simulink model "AmbhibiousDroneModel_tilt_mean"  (R2024b)
settings: Solver=FixedStepAuto  StartTime=0.0  StopTime=40  FixedStep=1/3000  RelTol=1e-3
model workspace (MAT data in the model file):
  Cd = 1.63886804e-09
  Ct = 6.43091818e-08
  Ixx = 113600
  Iyy = 113600
  Izz = 22620
  Lx = 0.133
  Ly = 0.1575
  Lz = 0.0132
  h = 0.05
  rho = 1.225
libraries: simulink_extras x10, slpidlib x3, aerolibanimutils x2, shared6dof x1, px4Sensorslib x1
settings Model: Creator=awahm  LastModifiedBy=Micheal Awah
settings RTWCC: GPUComputeCapability=3.5

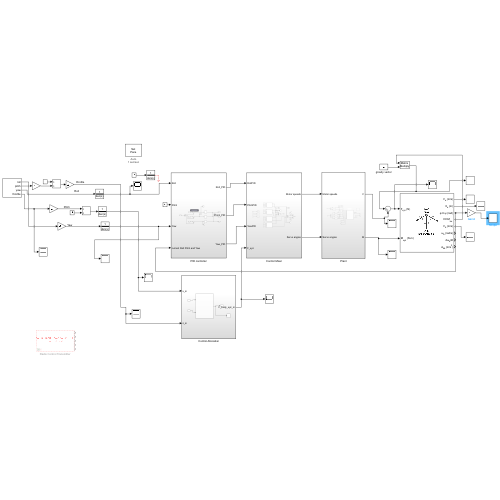
[thumbnail: Simulink's stored preview of the top-level diagram]
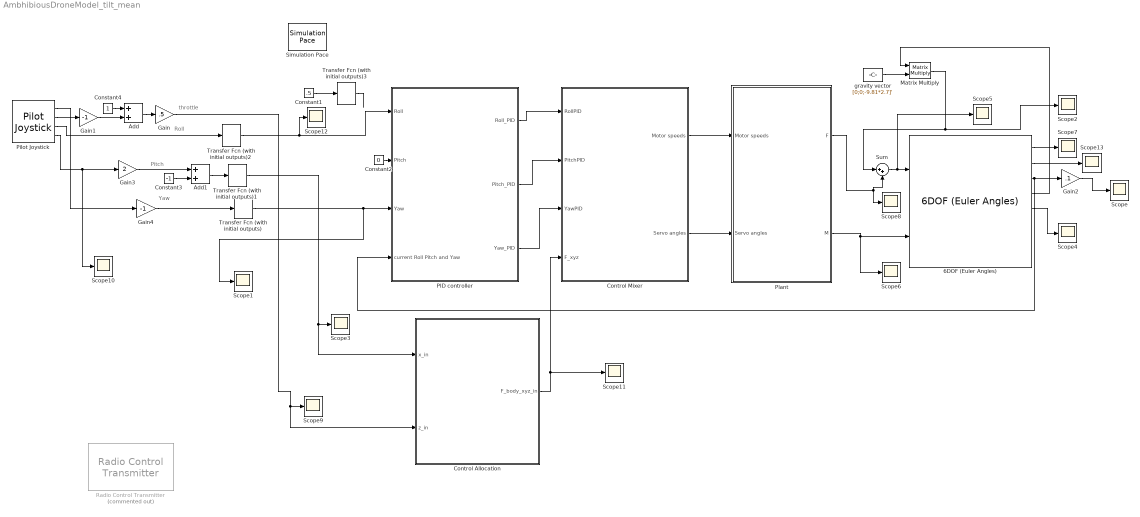
== system AmbhibiousDroneModel_tilt_mean ==
  note: throttle
  note: Roll
  note: Pitch
  note: Yaw
  6DOF (Euler Angles) : shared6dof/6DOF (Euler Angles)  units=Metric (MKS)  mtype=Fixed  rep=Euler Angles  xme_0=[0 0 0]  Vm_0=[0 0 0]  eul_0=[0 0 0]  pm_0=[0 0 0]  mass_0=7.2  mass_e=0.5  mass_f=2.0  inertia=[0.442 0 0;0 0.427 0; 0 0 0.659]  inertia_e=eye(3)  inertia_f=2*eye(3)  k_quat=1.0  vre_flag=on  abi_flag=off  aMode=0  xme_statename=''  Vm_statename=''  eul_statename=''  quat_statename=''  pm_statename=''  mass_statename=''
  Add : Sum
  Add1 : Sum
  Constant1 : Constant  Value=.5
  Constant2 : Constant  Value=0
  Constant3 : Constant  Value=-1
  Constant4 : Constant
  Control Allocation : Subsystem
  Control Mixer : Subsystem
  Gain : Gain  Gain=.5
  Gain1 : Gain  Gain=-1
  Gain2 : Gain  Gain=.1
  Gain3 : Gain  Gain=2
  Gain4 : Gain  Gain=-1
  Matrix Multiply : Product  Multiplication=Matrix(*)
  PID controller : Subsystem
  Pilot Joystick : aerolibanimutils/Pilot Joystick  JoystickID=Joystick1  OutputConfiguration=FourAxis  SampleTime=1/30
  Plant : Subsystem
  Radio Control Transmitter : px4Sensorslib/Radio Control Transmitter  Commented=on  channel1=on  channel2=on  channel3=on  channel4=on  channel5=off  channel6=off  channel7=off  channel8=off  channel_count=off  rssi=off  rc_input_source=off  timestamp_last_signal=off  time_stamp=off  sampleTime=1/250  BlockingMode=off  BlockTimeout=5
  Scope{,1..13} (14 alike) : Scope
  Simulation Pace : aerolibanimutils/Simulation Pace  SimulationPace=1  SleepMode=Auto  OutputPaceError=off  SampleTime=1/300
  Sum : Sum  Inputs=|++
  Transfer Fcn (with initial outputs){,1..3} (4 alike) : simulink_extras/Additional Linear/Transfer Fcn (with initial outputs)  N=[1]  D="[.25  1]"  Y0=0  U0=0
  gravity vector : Constant  Value=[0;0;-9.81*2.7]'
  wires:
  Plant/2(M) -> Scope6/1, 6DOF (Euler Angles)/2
  6DOF (Euler Angles)/4 -> Matrix Multiply/1
  gravity vector/1 -> Matrix Multiply/2
  Sum/1 -> Scope5/1, 6DOF (Euler Angles)/1
  6DOF (Euler Angles)/1 -> Scope7/1
  6DOF (Euler Angles)/5 -> Scope4/1
  Matrix Multiply/1 -> Sum/1, Scope2/1
  Pilot Joystick/1 -> Gain4/1
  PID controller/1(Roll_PID) -> Control Mixer/1(RollPID)
  PID controller/2(Pitch_PID) -> Control Mixer/2(PitchPID)
  PID controller/3(Yaw_PID) -> Control Mixer/3(YawPID)
  Control Mixer/1(Motor speeds) -> Plant/1(Motor speeds)
  Control Mixer/2(Servo angles) -> Plant/2(Servo angles)
  Plant/1(F) -> Sum/2, Scope8/1
  Pilot Joystick/4 -> Gain3/1, Scope10/1
  Pilot Joystick/3 -> Transfer Fcn (with initial outputs)2/1
  Pilot Joystick/2 -> Gain1/1
  Constant4/1 -> Add/1
  Add/1 -> Gain/1
  Gain1/1 -> Add/2
  Constant2/1 -> PID controller/2(Pitch)
  Constant1/1 -> Transfer Fcn (with initial outputs)3/1
  Gain3/1 -> Add1/1
  Constant3/1 -> Add1/2
  Add1/1 -> Transfer Fcn (with initial outputs)1/1
  Gain4/1 -> Transfer Fcn (with initial outputs)/1
  Transfer Fcn (with initial outputs)2/1 -> Scope12/1, PID controller/1(Roll)
  6DOF (Euler Angles)/3 -> Gain2/1, PID controller/4(current Roll Pitch and Yaw)
  Gain/1 -> Scope9/1, Control Allocation/2(z_in)
  Control Allocation/1(F_body_xyz_in) -> Control Mixer/4(F_xyz), Scope11/1
  Transfer Fcn (with initial outputs)/1 -> PID controller/3(Yaw), Scope1/1
  Transfer Fcn (with initial outputs)1/1 -> Control Allocation/1(x_in), Scope3/1
  Transfer Fcn (with initial outputs)3/1 -> ?
  6DOF (Euler Angles)/2 -> Scope13/1
  Gain2/1 -> Scope/1

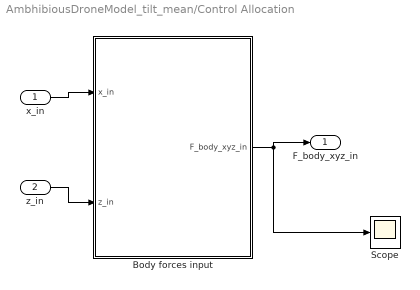
== system AmbhibiousDroneModel_tilt_mean/Control Allocation ==
  x_in : Inport
  z_in : Inport  Port=2
  Body forces input : MATLAB Function  TreatAsAtomicUnit=on
  Scope : Scope
  F_body_xyz_in : Outport
  wires:
  x_in/1 -> Body forces input/1(x_in)
  z_in/1 -> Body forces input/2(z_in)
  Body forces input/1(F_body_xyz_in) -> F_body_xyz_in/1, Scope/1

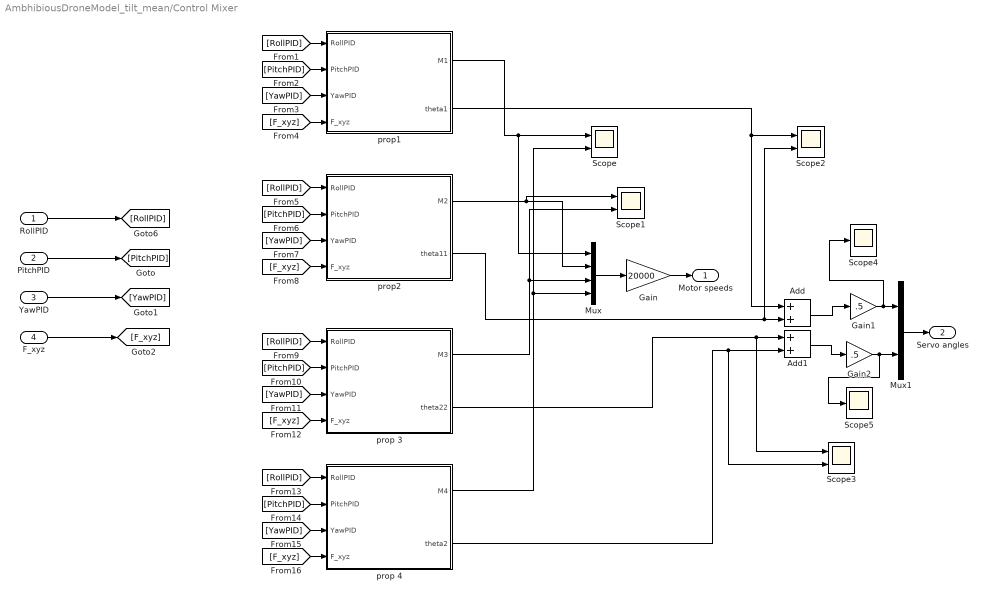
== system AmbhibiousDroneModel_tilt_mean/Control Mixer ==
  RollPID : Inport
  PitchPID : Inport  Port=2
  YawPID : Inport  Port=3
  F_xyz : Inport  Port=4
  Add : Sum
  Add1 : Sum
  Gain : Gain  Gain=20000
  Gain1 : Gain  Gain=.5
  Gain2 : Gain  Gain=.5
  Mux : Mux
  Mux1 : Mux  Inputs=2
  Scope{,1..3} (4 alike) : Scope  NumInputPorts=2
  Scope4 : Scope
  Scope5 : Scope
  prop 3 : Subsystem
  prop 4 : Subsystem
  "prop1 " : Subsystem
  prop2 : Subsystem
  Motor speeds : Outport
  Servo angles : Outport  Port=2
  wires:
  "prop1 "/1(M1) -> Mux/1, Scope/1
  PitchPID/1 -> [PitchPID]
  YawPID/1 -> [YawPID]
  RollPID/1 -> [RollPID]
  [F_xyz] -> "prop1 "/4(F_xyz)
  [YawPID] -> "prop1 "/3(YawPID)
  [PitchPID] -> "prop1 "/2(PitchPID)
  [RollPID] -> "prop1 "/1(RollPID)
  prop2/1(M2) -> Mux/2, Scope1/1
  prop 4/2(theta2) -> Scope3/2, Add1/2
  prop 3/1(M3) -> Scope1/2, Mux/3
  prop 4/1(M4) -> Scope/2, Mux/4
  Mux/1 -> Gain/1
  Mux1/1 -> Servo angles/1
  Gain/1 -> Motor speeds/1
  F_xyz/1 -> [F_xyz]
  [RollPID] -> prop2/1(RollPID)
  [PitchPID] -> prop2/2(PitchPID)
  [YawPID] -> prop2/3(YawPID)
  [F_xyz] -> prop2/4(F_xyz)
  [RollPID] -> prop 3/1(RollPID)
  [PitchPID] -> prop 3/2(PitchPID)
  [YawPID] -> prop 3/3(YawPID)
  [F_xyz] -> prop 3/4(F_xyz)
  [RollPID] -> prop 4/1(RollPID)
  [PitchPID] -> prop 4/2(PitchPID)
  [YawPID] -> prop 4/3(YawPID)
  [F_xyz] -> prop 4/4(F_xyz)
  Gain1/1 -> Scope4/1, Mux1/1
  Gain2/1 -> Scope5/1, Mux1/2
  Add/1 -> Gain1/1
  prop 3/2(theta22) -> Scope3/1, Add1/1
  prop2/2(theta11) -> Scope2/2, Add/2
  "prop1 "/2(theta1) -> Scope2/1, Add/1
  Add1/1 -> Gain2/1

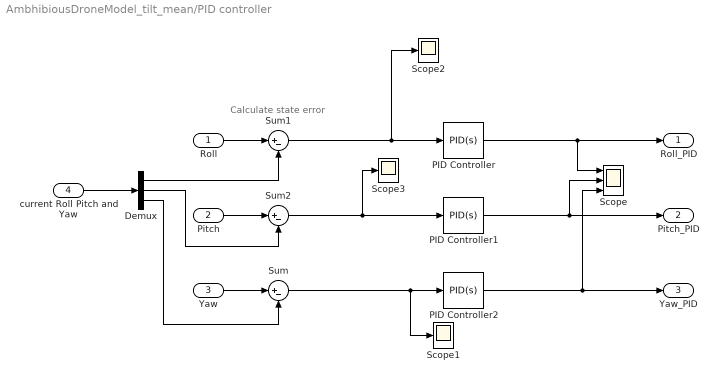
== system AmbhibiousDroneModel_tilt_mean/PID controller ==
  note: Calculate state error
  Roll : Inport
  Pitch : Inport  Port=2
  Yaw : Inport  Port=3
  current Roll Pitch and Yaw : Inport  Port=4
  Demux : Demux  Outputs=3
  PID Controller : slpidlib/PID Controller  Controller=PID  Form=Parallel  TimeDomain=Continuous-time  UseExternalTs=off  SampleTime=-1  IntegratorMethod=Forward Euler  FilterMethod=Forward Euler  ControllerParametersSource=internal  P=.2  I=.3  UseKiTs=off  D=.1  UseExternalDerivativeSource=off  N=100  UseFilter=on  TunerSelectOption=Transfer Function Based (PID Tuner App)  InitialConditionSource=internal  InitialConditionForIntegrator=0  InitialConditionForFilter=0  DifferentiatorICPrevScaledInput=0  ExternalReset=none  TrackingMode=off  Kt=1  LimitOutput=off  SatLimitsSource=internal  UpperSaturationLimit=inf  LowerSaturationLimit=-inf  LinearizeAsGain=on  AntiWindupMode=none  Kb=1  LimitIntegrator=off  UpperIntegratorSaturationLimit=inf  LowerIntegratorSaturationLimit=-inf  POutMin=[]  POutMax=[]  IOutMin=[]  IOutMax=[]  DOutMin=[]  DOutMax=[]  NOutMin=[]  NOutMax=[]  SumOutMin=[]  SumOutMax=[]  SaturationOutMin=[]  SaturationOutMax=[]  PParamMin=[]  PParamMax=[]  IParamMin=[]  IParamMax=[]  DParamMin=[]  DParamMax=[]  NParamMin=[]  NParamMax=[]  KbParamMin=[]  KbParamMax=[]  KtParamMin=[]  KtParamMax=[]  KbOutMin=[]  KbOutMax=[]  KtOutMin=[]  KtOutMax=[]  IntegratorOutMin=[]  IntegratorOutMax=[]  FilterOutMin=[]  FilterOutMax=[]  SumI1OutMin=[]  SumI1OutMax=[]  SumI2OutMin=[]  SumI2OutMax=[]  SumI3OutMin=[]  SumI3OutMax=[]  SumI4OutMin=[]  SumI4OutMax=[]  SumDOutMin=[]  SumDOutMax=[]  DifferentiatorOutMin=[]  DifferentiatorOutMax=[]  FilterDiffOutCoefMin=[]  FilterDiffOutCoefMax=[]  ReciprocalOutMin=[]  ReciprocalOutMax=[]  SumDenOutMin=[]  SumDenOutMax=[]  SumNumOutMin=[]  SumNumOutMax=[]  DivideOutMin=[]  DivideOutMax=[]  UdiffTsProdOutMin=[]  UdiffTsProdOutMax=[]  NTsProdOutMin=[]  NTsProdOutMax=[]  UintegralTsProdOutMin=[]  UintegralTsProdOutMax=[]  UngainTsProdOutMin=[]  UngainTsProdOutMax=[]  ClampingZeroOutDataTypeStr=Inherit: Inherit via back propagation  ClampingZeroOutMin=[]  ClampingZeroOutMax=[]  FilterDenConstantOutDataTypeStr=Inherit: Inherit via back propagation  FilterDenConstantOutMin=[]  FilterDenConstantOutMax=[]  PCopyOutDataTypeStr=Inherit: Inherit via back propagation  PCopyOutMin=[]  PCopyOutMax=[]  NCopyOutDataTypeStr=Inherit: Inherit via back propagation  NCopyOutMin=[]  NCopyOutMax=[]  IntegratorContinuousStateAttributes=''  IntegratorStateMustResolveToSignalObject=off  IntegratorRTWStateStorageClass=Auto  FilterContinuousStateAttributes=''  FilterStateMustResolveToSignalObject=off  FilterRTWStateStorageClass=Auto  ParallelPVariant=InternalParameters  IdealPVariant=Disabled  IVariant=InternalParameters  DVariant=InternalParameters  IntegratorVariant=Continuous  SatVariant=Disabled  AWVariant=Passthrough  PCopyVariant=Disabled  TRVariant=Disabled  FdbkBlocksVariant=Forward  IdealPFdbkVariant=Disabled  SatFdbkVariant=Disabled  DerivativeFilterVariant=ContFilter  NVariant=InternalParameters  NCopyVariant=Disabled  FilterICVariant=InternalICsFilter  IntegratorICVariant=InternalICs  ExternalResetVariant=Disabled  TRSumVariant=Passthrough  SumFdbkVariant=Disabled  SumVariant=Sum_PID  TsampFilterVariant=InternalTs  TsampNgainVariant=Passthrough  TsampIntegralVariant=Disabled_SignalSpec  ExternalSaturationOutDataTypeStr=Inherit: Same as second input  DerivativeSourceVariant=ErrorSignal  PreIntVariant=InternalPreInt
  PID Controller1 : slpidlib/PID Controller  Controller=PID  Form=Parallel  TimeDomain=Continuous-time  UseExternalTs=off  SampleTime=-1  IntegratorMethod=Forward Euler  FilterMethod=Forward Euler  ControllerParametersSource=internal  P=.2  I=.3  UseKiTs=off  D=.1  UseExternalDerivativeSource=off  N=100  UseFilter=on  TunerSelectOption=Transfer Function Based (PID Tuner App)  InitialConditionSource=internal  InitialConditionForIntegrator=0  InitialConditionForFilter=0  DifferentiatorICPrevScaledInput=0  ExternalReset=none  TrackingMode=off  Kt=1  LimitOutput=off  SatLimitsSource=internal  UpperSaturationLimit=inf  LowerSaturationLimit=-inf  LinearizeAsGain=on  AntiWindupMode=none  Kb=1  LimitIntegrator=off  UpperIntegratorSaturationLimit=inf  LowerIntegratorSaturationLimit=-inf  POutMin=[]  POutMax=[]  IOutMin=[]  IOutMax=[]  DOutMin=[]  DOutMax=[]  NOutMin=[]  NOutMax=[]  SumOutMin=[]  SumOutMax=[]  SaturationOutMin=[]  SaturationOutMax=[]  PParamMin=[]  PParamMax=[]  IParamMin=[]  IParamMax=[]  DParamMin=[]  DParamMax=[]  NParamMin=[]  NParamMax=[]  KbParamMin=[]  KbParamMax=[]  KtParamMin=[]  KtParamMax=[]  KbOutMin=[]  KbOutMax=[]  KtOutMin=[]  KtOutMax=[]  IntegratorOutMin=[]  IntegratorOutMax=[]  FilterOutMin=[]  FilterOutMax=[]  SumI1OutMin=[]  SumI1OutMax=[]  SumI2OutMin=[]  SumI2OutMax=[]  SumI3OutMin=[]  SumI3OutMax=[]  SumI4OutMin=[]  SumI4OutMax=[]  SumDOutMin=[]  SumDOutMax=[]  DifferentiatorOutMin=[]  DifferentiatorOutMax=[]  FilterDiffOutCoefMin=[]  FilterDiffOutCoefMax=[]  ReciprocalOutMin=[]  ReciprocalOutMax=[]  SumDenOutMin=[]  SumDenOutMax=[]  SumNumOutMin=[]  SumNumOutMax=[]  DivideOutMin=[]  DivideOutMax=[]  UdiffTsProdOutMin=[]  UdiffTsProdOutMax=[]  NTsProdOutMin=[]  NTsProdOutMax=[]  UintegralTsProdOutMin=[]  UintegralTsProdOutMax=[]  UngainTsProdOutMin=[]  UngainTsProdOutMax=[]  ClampingZeroOutDataTypeStr=Inherit: Inherit via back propagation  ClampingZeroOutMin=[]  ClampingZeroOutMax=[]  FilterDenConstantOutDataTypeStr=Inherit: Inherit via back propagation  FilterDenConstantOutMin=[]  FilterDenConstantOutMax=[]  PCopyOutDataTypeStr=Inherit: Inherit via back propagation  PCopyOutMin=[]  PCopyOutMax=[]  NCopyOutDataTypeStr=Inherit: Inherit via back propagation  NCopyOutMin=[]  NCopyOutMax=[]  IntegratorContinuousStateAttributes=''  IntegratorStateMustResolveToSignalObject=off  IntegratorRTWStateStorageClass=Auto  FilterContinuousStateAttributes=''  FilterStateMustResolveToSignalObject=off  FilterRTWStateStorageClass=Auto  ParallelPVariant=InternalParameters  IdealPVariant=Disabled  IVariant=InternalParameters  DVariant=InternalParameters  IntegratorVariant=Continuous  SatVariant=Disabled  AWVariant=Passthrough  PCopyVariant=Disabled  TRVariant=Disabled  FdbkBlocksVariant=Forward  IdealPFdbkVariant=Disabled  SatFdbkVariant=Disabled  DerivativeFilterVariant=ContFilter  NVariant=InternalParameters  NCopyVariant=Disabled  FilterICVariant=InternalICsFilter  IntegratorICVariant=InternalICs  ExternalResetVariant=Disabled  TRSumVariant=Passthrough  SumFdbkVariant=Disabled  SumVariant=Sum_PID  TsampFilterVariant=InternalTs  TsampNgainVariant=Passthrough  TsampIntegralVariant=Disabled_SignalSpec  ExternalSaturationOutDataTypeStr=Inherit: Same as second input  DerivativeSourceVariant=ErrorSignal  PreIntVariant=InternalPreInt
  PID Controller2 : slpidlib/PID Controller  Controller=PID  Form=Parallel  TimeDomain=Continuous-time  UseExternalTs=off  SampleTime=-1  IntegratorMethod=Forward Euler  FilterMethod=Forward Euler  ControllerParametersSource=internal  P=.2  I=.1  UseKiTs=off  D=.35  UseExternalDerivativeSource=off  N=100  UseFilter=on  TunerSelectOption=Transfer Function Based (PID Tuner App)  InitialConditionSource=internal  InitialConditionForIntegrator=0  InitialConditionForFilter=0  DifferentiatorICPrevScaledInput=0  ExternalReset=none  TrackingMode=off  Kt=1  LimitOutput=off  SatLimitsSource=internal  UpperSaturationLimit=inf  LowerSaturationLimit=-inf  LinearizeAsGain=on  AntiWindupMode=none  Kb=1  LimitIntegrator=off  UpperIntegratorSaturationLimit=inf  LowerIntegratorSaturationLimit=-inf  POutMin=[]  POutMax=[]  IOutMin=[]  IOutMax=[]  DOutMin=[]  DOutMax=[]  NOutMin=[]  NOutMax=[]  SumOutMin=[]  SumOutMax=[]  SaturationOutMin=[]  SaturationOutMax=[]  PParamMin=[]  PParamMax=[]  IParamMin=[]  IParamMax=[]  DParamMin=[]  DParamMax=[]  NParamMin=[]  NParamMax=[]  KbParamMin=[]  KbParamMax=[]  KtParamMin=[]  KtParamMax=[]  KbOutMin=[]  KbOutMax=[]  KtOutMin=[]  KtOutMax=[]  IntegratorOutMin=[]  IntegratorOutMax=[]  FilterOutMin=[]  FilterOutMax=[]  SumI1OutMin=[]  SumI1OutMax=[]  SumI2OutMin=[]  SumI2OutMax=[]  SumI3OutMin=[]  SumI3OutMax=[]  SumI4OutMin=[]  SumI4OutMax=[]  SumDOutMin=[]  SumDOutMax=[]  DifferentiatorOutMin=[]  DifferentiatorOutMax=[]  FilterDiffOutCoefMin=[]  FilterDiffOutCoefMax=[]  ReciprocalOutMin=[]  ReciprocalOutMax=[]  SumDenOutMin=[]  SumDenOutMax=[]  SumNumOutMin=[]  SumNumOutMax=[]  DivideOutMin=[]  DivideOutMax=[]  UdiffTsProdOutMin=[]  UdiffTsProdOutMax=[]  NTsProdOutMin=[]  NTsProdOutMax=[]  UintegralTsProdOutMin=[]  UintegralTsProdOutMax=[]  UngainTsProdOutMin=[]  UngainTsProdOutMax=[]  ClampingZeroOutDataTypeStr=Inherit: Inherit via back propagation  ClampingZeroOutMin=[]  ClampingZeroOutMax=[]  FilterDenConstantOutDataTypeStr=Inherit: Inherit via back propagation  FilterDenConstantOutMin=[]  FilterDenConstantOutMax=[]  PCopyOutDataTypeStr=Inherit: Inherit via back propagation  PCopyOutMin=[]  PCopyOutMax=[]  NCopyOutDataTypeStr=Inherit: Inherit via back propagation  NCopyOutMin=[]  NCopyOutMax=[]  IntegratorContinuousStateAttributes=''  IntegratorStateMustResolveToSignalObject=off  IntegratorRTWStateStorageClass=Auto  FilterContinuousStateAttributes=''  FilterStateMustResolveToSignalObject=off  FilterRTWStateStorageClass=Auto  ParallelPVariant=InternalParameters  IdealPVariant=Disabled  IVariant=InternalParameters  DVariant=InternalParameters  IntegratorVariant=Continuous  SatVariant=Disabled  AWVariant=Passthrough  PCopyVariant=Disabled  TRVariant=Disabled  FdbkBlocksVariant=Forward  IdealPFdbkVariant=Disabled  SatFdbkVariant=Disabled  DerivativeFilterVariant=ContFilter  NVariant=InternalParameters  NCopyVariant=Disabled  FilterICVariant=InternalICsFilter  IntegratorICVariant=InternalICs  ExternalResetVariant=Disabled  TRSumVariant=Passthrough  SumFdbkVariant=Disabled  SumVariant=Sum_PID  TsampFilterVariant=InternalTs  TsampNgainVariant=Passthrough  TsampIntegralVariant=Disabled_SignalSpec  ExternalSaturationOutDataTypeStr=Inherit: Same as second input  DerivativeSourceVariant=ErrorSignal  PreIntVariant=InternalPreInt
  Scope : Scope  NumInputPorts=3
  Scope1 : Scope
  Scope2 : Scope
  Scope3 : Scope
  Sum : Sum  Inputs=|+-
  Sum1 : Sum  Inputs=|+-
  Sum2 : Sum  Inputs=|+-
  Roll_PID : Outport
  Pitch_PID : Outport  Port=2
  Yaw_PID : Outport  Port=3
  wires:
  Demux/3 -> Sum/2
  Demux/2 -> Sum2/2
  Demux/1 -> Sum1/2
  current Roll Pitch and Yaw/1 -> Demux/1
  Sum/1 -> Scope1/1, PID Controller2/1
  Roll/1 -> Sum1/1
  Pitch/1 -> Sum2/1
  Yaw/1 -> Sum/1
  Sum1/1 -> Scope2/1, PID Controller/1
  Sum2/1 -> Scope3/1, PID Controller1/1
  PID Controller/1 -> Roll_PID/1, Scope/1
  PID Controller2/1 -> Yaw_PID/1, Scope/3
  PID Controller1/1 -> Pitch_PID/1, Scope/2

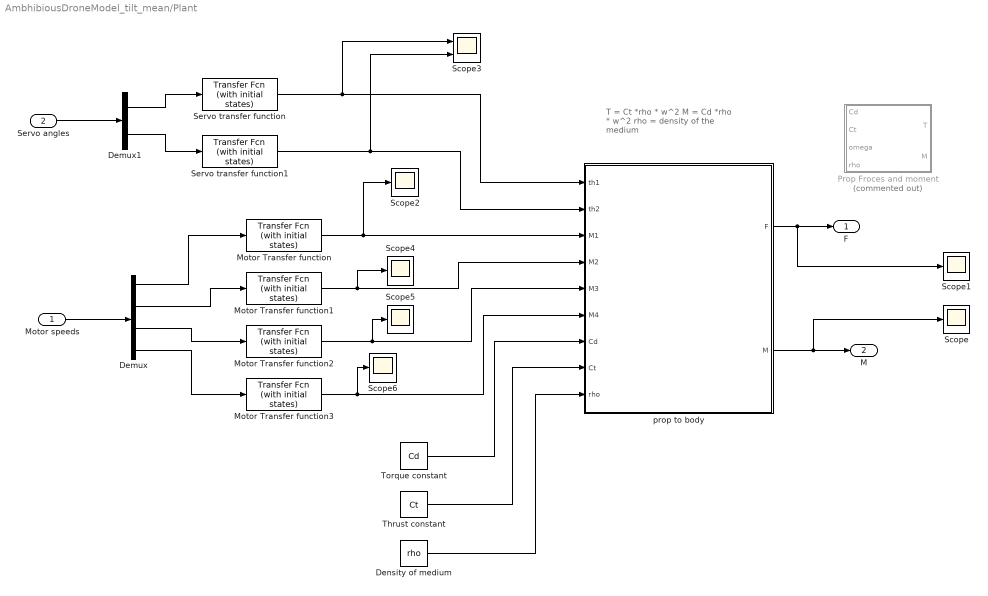
== system AmbhibiousDroneModel_tilt_mean/Plant ==
  note: T = Ct *rho * w^2
      | M = Cd *rho * w^2
      | rho = density of the medium
  Motor speeds : Inport
  Servo angles : Inport  Port=2
  Demux : Demux
  Demux1 : Demux  Outputs=2
  Density of medium : Constant  Value=rho
  Motor Transfer function{,1..3} (4 alike) : simulink_extras/Additional Linear/Transfer Fcn (with initial states)  N=[153.35]  D=[1 20.06 153.35]  X0=0
  Prop Froces and moment : Subsystem  Commented=on
  Scope{,1..2,4..6} (6 alike) : Scope
  Scope3 : Scope  NumInputPorts=2
  Servo transfer function : simulink_extras/Additional Linear/Transfer Fcn (with initial states)  N=[153.35]  D=[1 20.06 153.35]  X0=0
  Servo transfer function1 : simulink_extras/Additional Linear/Transfer Fcn (with initial states)  N=[153.35]  D=[1 20.06 153.35]  X0=0
  Thrust constant : Constant  Value=Ct
  Torque constant : Constant  Value=Cd
  prop to body : MATLAB Function  TreatAsAtomicUnit=on
  F : Outport
  M : Outport  Port=2
  wires:
  Motor speeds/1 -> Demux/1
  Servo angles/1 -> Demux1/1
  Demux/3 -> Motor Transfer function2/1
  Demux/4 -> Motor Transfer function3/1
  Demux1/1 -> Servo transfer function/1
  Demux1/2 -> Servo transfer function1/1
  Demux/1 -> Motor Transfer function/1
  Demux/2 -> Motor Transfer function1/1
  Thrust constant/1 -> prop to body/8(Ct)
  prop to body/1(F) -> Scope1/1, F/1
  Torque constant/1 -> prop to body/7(Cd)
  Motor Transfer function/1 -> Scope2/1, prop to body/3(M1)
  Density of medium/1 -> prop to body/9(rho)
  Motor Transfer function1/1 -> Scope4/1, prop to body/4(M2)
  Motor Transfer function2/1 -> Scope5/1, prop to body/5(M3)
  Motor Transfer function3/1 -> Scope6/1, prop to body/6(M4)
  Servo transfer function1/1 -> Scope3/2, prop to body/2(th2)
  prop to body/2(M) -> Scope/1, M/1
  Servo transfer function/1 -> Scope3/1, prop to body/1(th1)

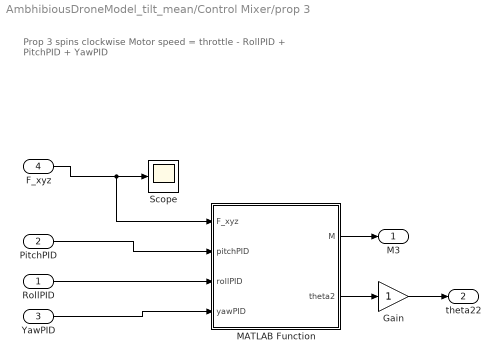
== system AmbhibiousDroneModel_tilt_mean/Control Mixer/prop 3 ==
  note: Prop 3 spins clockwise
      | Motor speed = throttle - RollPID + PitchPID + YawPID
  RollPID : Inport
  PitchPID : Inport  Port=2
  YawPID : Inport  Port=3
  F_xyz : Inport  Port=4
  Gain : Gain
  MATLAB Function : MATLAB Function  TreatAsAtomicUnit=on
  Scope : Scope
  M3 : Outport
  theta22 : Outport  Port=2
  wires:
  YawPID/1 -> MATLAB Function/4(yawPID)
  F_xyz/1 -> MATLAB Function/1(F_xyz), Scope/1
  RollPID/1 -> MATLAB Function/3(rollPID)
  MATLAB Function/1(M) -> M3/1
  MATLAB Function/2(theta2) -> Gain/1
  PitchPID/1 -> MATLAB Function/2(pitchPID)
  Gain/1 -> theta22/1

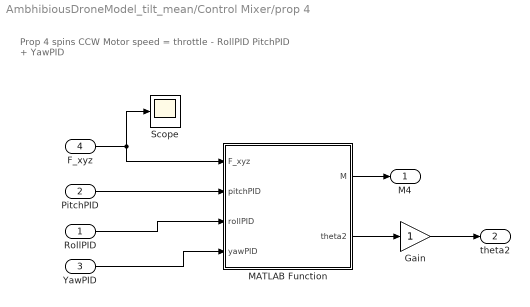
== system AmbhibiousDroneModel_tilt_mean/Control Mixer/prop 4 ==
  note: Prop 4 spins CCW
      | Motor speed = throttle - RollPID   PitchPID + YawPID
  RollPID : Inport
  PitchPID : Inport  Port=2
  YawPID : Inport  Port=3
  F_xyz : Inport  Port=4
  Gain : Gain
  MATLAB Function : MATLAB Function  TreatAsAtomicUnit=on
  Scope : Scope
  M4 : Outport
  theta2 : Outport  Port=2
  wires:
  YawPID/1 -> MATLAB Function/4(yawPID)
  F_xyz/1 -> Scope/1, MATLAB Function/1(F_xyz)
  RollPID/1 -> MATLAB Function/3(rollPID)
  PitchPID/1 -> MATLAB Function/2(pitchPID)
  MATLAB Function/1(M) -> M4/1
  MATLAB Function/2(theta2) -> Gain/1
  Gain/1 -> theta2/1

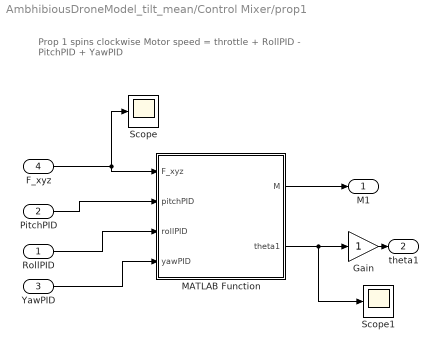
== system AmbhibiousDroneModel_tilt_mean/Control Mixer/prop1  ==
  note: Prop 1 spins clockwise
      | Motor speed = throttle + RollPID - PitchPID + YawPID
  RollPID : Inport
  PitchPID : Inport  Port=2
  YawPID : Inport  Port=3
  F_xyz : Inport  Port=4
  Gain : Gain
  MATLAB Function : MATLAB Function  TreatAsAtomicUnit=on
  Scope : Scope
  Scope1 : Scope
  M1 : Outport
  theta1 : Outport  Port=2
  wires:
  MATLAB Function/2(theta1) -> Scope1/1, Gain/1
  F_xyz/1 -> Scope/1, MATLAB Function/1(F_xyz)
  RollPID/1 -> MATLAB Function/3(rollPID)
  PitchPID/1 -> MATLAB Function/2(pitchPID)
  YawPID/1 -> MATLAB Function/4(yawPID)
  MATLAB Function/1(M) -> M1/1
  Gain/1 -> theta1/1

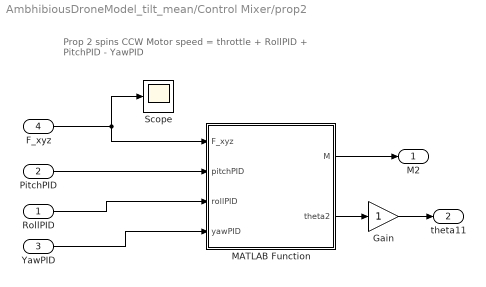
== system AmbhibiousDroneModel_tilt_mean/Control Mixer/prop2 ==
  note: Prop 2 spins CCW
      | Motor speed = throttle + RollPID + PitchPID - YawPID
  RollPID : Inport
  PitchPID : Inport  Port=2
  YawPID : Inport  Port=3
  F_xyz : Inport  Port=4
  Gain : Gain
  MATLAB Function : MATLAB Function  TreatAsAtomicUnit=on
  Scope : Scope
  M2 : Outport
  theta11 : Outport  Port=2
  wires:
  YawPID/1 -> MATLAB Function/4(yawPID)
  F_xyz/1 -> Scope/1, MATLAB Function/1(F_xyz)
  RollPID/1 -> MATLAB Function/3(rollPID)
  PitchPID/1 -> MATLAB Function/2(pitchPID)
  MATLAB Function/1(M) -> M2/1
  MATLAB Function/2(theta2) -> Gain/1
  Gain/1 -> theta11/1

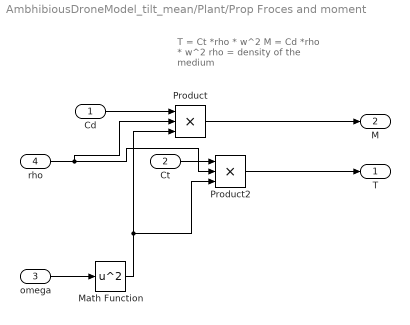
== system AmbhibiousDroneModel_tilt_mean/Plant/Prop Froces and moment ==
  note: T = Ct *rho * w^2
      | M = Cd *rho * w^2
      | rho = density of the medium
  Cd : Inport
  Ct : Inport  Port=2
  omega : Inport  Port=3
  rho : Inport  Port=4
  Math Function : Math  Operator=square
  Product : Product  Inputs=3
  Product2 : Product  Inputs=3
  T : Outport
  M : Outport  Port=2
  wires:
  omega/1 -> Math Function/1
  Ct/1 -> Product2/1
  Product2/1 -> T/1
  Product/1 -> M/1
  Cd/1 -> Product/1
  Math Function/1 -> Product2/3, Product/3
  rho/1 -> Product/2, Product2/2

== matlab function AmbhibiousDroneModel_tilt_mean/Plant/prop to body ==
  data: th1 input; F output; th2 input; M1 input; M2 input; M3 input; M4 input; Cd input; Ct input; rho input; M output
function [F,M] = fcn(th1,th2,M1,M2,M3,M4,Cd,Ct,rho)

T1 = Ct*rho*M1^2;
T2 = Ct*rho*M2^2;
T3 = Ct*rho*M3^2;
T4 = Ct*rho*M4^2;

C = Cd/Ct;

Ly = 0.133;
Lx = 0.1575;
d = -0.0132;

y = [Ly*T1*cos(th1) - Ly*T2*cos(th1) - Ly*T3*cos(th2) + Ly*T4*cos(th2) - C*T1*sin(th1) + C*T2*sin(th1) - C*T3*sin(th2) + C*T4*sin(th2);
     T3*(Lx*cos(th2) + d*sin(th2)) - T2*(Lx*cos(th1) - d*sin(th1)) - T1*(Lx*cos(th1) - d*sin(th1)) + T4*(Lx*cos(th2) + d*sin(th2));
     C*T2*cos(th1) - C*T1*cos(th1) - C*T3*cos(th2) + C*T4*cos(th2) - Ly*T1*sin(th1) + Ly*T2*sin(th1) + Ly*T3*sin(th2) - Ly*T4*sin(th2);
                                                                            T1*sin(th1) + T2*sin(th1) + T3*sin(th2) + T4*sin(th2);
                                                                                                                                0;
                                                                            T1*cos(th1) + T2*cos(th1) + T3*cos(th2) + T4*cos(th2)];
M = y(1:3);
F = y(4:6);

== matlab function AmbhibiousDroneModel_tilt_mean/Control Allocation/Body forces input ==
  data: x_in input; F_body_xyz_in output; z_in input
function F_body_xyz_in = fcn(x_in, z_in)
g = 9.81;
mass = 2.7;
V_cap = [x_in;0;z_in];  
F_body_xyz_in = V_cap;

% if z_in >= 0.5
%     % Define the input range
%     input_min = 0.5;
%     input_max = 1;
% 
%     % Define the output range
%     % output_min = 0;
%     output_max = 20; %making upward vertical acceleration
% 
%     % Map the input value to the output range
%     output_value = ((z_in - input_min) / (input_max - input_min)) * (output_max - output_min) + output_min;
% else
%     % Define the input range
%     input_min = 0;
%     input_max = 0.5;
% 
%     % Define the output range
%     output_min = -5; %max possible downward acceleration
%     output_max = 0;
% 
%     % Map the input value to the output range
%     output_value = ((z_in - input_min) / (input_max - input_min)) * (output_max - output_min) + output_min;
% end
% 
% F_body_xyz_in(3) = F_body_xyz_in(3) + output_value*mass; %adding acceleration due to throttle
% 
% deno = sqrt(F_body_xyz_in(3)^2 + F_body_xyz_in(1)^2);  %to use for norm, not that y-comp is not effective
% F_body_xyz_in = F_body_xyz_in/deno;  %normalizing

== matlab function AmbhibiousDroneModel_tilt_mean/Control Mixer/prop1 /MATLAB Function ==
  data: F_xyz input; pitchPID input; M output; theta1 output; rollPID input; yawPID input
function [M,theta1] = fcn(F_xyz, pitchPID, rollPID, yawPID)

fx = F_xyz(1) - yawPID;  %yaw control
fz = F_xyz(3) - pitchPID + rollPID;  %pitch and roll control

M = sqrt(fx^2 + fz^2);  %resultant force is simply the thust

%angles need to be tuned correctly to form a full cricle. 
theta1 = atan2(fx, fz);  % Compute angle in radians, range is -pi to pi
if theta1 < 0
    theta1 = theta1 + 2*pi;  % Adjust to range 0 to 2*pi
end

% Check if theta1 is close to zero (within -1 to 0 degrees) and set it to zero
if theta1 > 2*pi - deg2rad(10)  % Convert -1 degree to radians and check
    theta1 = 0;
end

== matlab function AmbhibiousDroneModel_tilt_mean/Control Mixer/prop 4/MATLAB Function ==
  data: F_xyz input; pitchPID input; M output; theta2 output; rollPID input; yawPID input
function [M,theta2] = fcn(F_xyz, pitchPID, rollPID, yawPID)

fx = F_xyz(1) - yawPID;  %yaw control
fz = F_xyz(3) + pitchPID + rollPID;  %pitch and roll control

M = sqrt(fx^2 + fz^2);  %resultant force is simply the thust


%angles need to be tuned correctly to form a full cricle. 
theta2 = atan2(fx, fz);  % Compute angle in radians, range is -pi to pi
if theta2 < 0
    theta2 = theta2 + 2*pi;  % Adjust to range 0 to 2*pi
end

% Check if theta1 is close to zero (within -1 to 0 degrees) and set it to zero
if theta2 > 2*pi - deg2rad(10)  % Convert -1 degree to radians and check
    theta2 = 0;
end

== matlab function AmbhibiousDroneModel_tilt_mean/Control Mixer/prop2/MATLAB Function ==
  data: F_xyz input; pitchPID input; M output; theta2 output; rollPID input; yawPID input
function [M,theta2] = fcn(F_xyz, pitchPID, rollPID, yawPID)

fx = F_xyz(1) + yawPID;  %yaw control
fz = F_xyz(3) - pitchPID - rollPID;  %pitch and roll control

M = sqrt(fx^2 + fz^2);  %resultant force is simply the thust


%angles need to be tuned correctly to form a full cricle. 
theta2 = atan2(fx, fz);  % Compute angle in radians, range is -pi to pi
if theta2 < 0
    theta2 = theta2 + 2*pi;  % Adjust to range 0 to 2*pi
end

% Check if theta1 is close to zero (within -1 to 0 degrees) and set it to zero
if theta2 > 2*pi - deg2rad(10)  % Convert -1 degree to radians and check
    theta2 = 0;
end

== matlab function AmbhibiousDroneModel_tilt_mean/Control Mixer/prop 3/MATLAB Function ==
  data: F_xyz input; pitchPID input; M output; theta2 output; rollPID input; yawPID input
function [M,theta2] = fcn(F_xyz, pitchPID, rollPID, yawPID)

fx = F_xyz(1) + yawPID;  %yaw control
fz = F_xyz(3) + pitchPID - rollPID;  %pitch and roll control

M = sqrt(fx^2 + fz^2);  %resultant force is simply the thust


%angles need to be tuned correctly to form a full cricle. 
theta2 = atan2(fx, fz);  % Compute angle in radians, range is -pi to pi
if theta2 < 0
    theta2 = theta2 + 2*pi;  % Adjust to range 0 to 2*pi
end

% Check if theta1 is close to zero (within -1 to 0 degrees) and set it to zero
if theta2 > 2*pi - deg2rad(10)  % Convert -1 degree to radians and check
    theta2 = 0;
end
